simulink model "Filter_design"  (R2014a)
settings: Solver=ode45  StartTime=0.0  StopTime=10.0  RelTol=1e-3
settings Model: Creator=Iseberg-2  LastModifiedBy=Iseberg-2

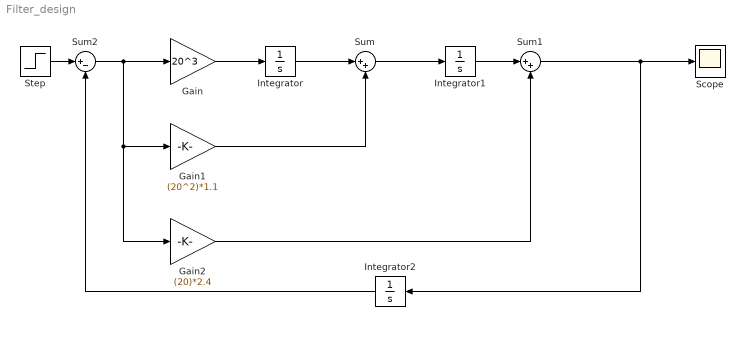
== system Filter_design ==
  Gain : Gain  Gain=20^3
  Gain1 : Gain  Gain=(20^2)*1.1
  Gain2 : Gain  Gain=(20)*2.4
  Integrator : Integrator
  Integrator1 : Integrator
  Integrator2 : Integrator
  Scope : Scope
      settings: TimeRange=4  YMin=0.7721088435374153  YMax=4.772108843537415
  Step : Step  SampleTime=0
  Sum : Sum  Inputs=|++
  Sum1 : Sum  Inputs=|++
  Sum2 : Sum  Inputs=|+-
  wires:
  Gain/1 -> Integrator/1
  Integrator/1 -> Sum/1
  Gain1/1 -> Sum/2
  Sum/1 -> Integrator1/1
  Integrator1/1 -> Sum1/1
  Gain2/1 -> Sum1/2
  Sum2/1 -> Gain2/1, Gain1/1, Gain/1
  Sum1/1 -> Scope/1, Integrator2/1
  Step/1 -> Sum2/1
  Integrator2/1 -> Sum2/2
